simulink model "DahldissertacaoJoao"  (R2017a)
settings: Solver=ode3  StartTime=0.0  StopTime=max(Time)  FixedStep=dt  RelTol=1e-3  EnableMultiTasking=on
values from neighbouring files (symbols this model uses):
  Kw = 57.42    [maincode.m]
  Kx = 0.7682    [maincode.m]
  n = 1    [maincode.m]
  rho = 27.45    [maincode.m]
settings Model: Creator=Administrador  LastModifiedBy=vargas
settings DataIOCC: LimitDataPoints=on  SaveFormat=Array  SignalLoggingSaveFormat=ModelDataLogs
settings OptimizationCC: ExpressionDepthLimit=2147483647  LifeSpan=inf
settings DebuggingCC: UnderspecifiedInitializationDetection=Classic  MergeDetectMultiDrivingBlocksExec=none  SolverPrmCheckMsg=warning  FcnCallInpInsideContextMsg=warning  StateNameClashWarn=warning  SFUnexpectedBacktrackingDiag=warning  SFNoUnconditionalDefaultTransitionDiag=warning  SFExecutionAtInitializationDiag=none
settings HardwareCC: ProdBitPerPointer=32  ProdBitPerSizeT=32  ProdBitPerPtrDiffT=32  ProdLargestAtomicFloat=None  ProdIntDivRoundTo=Undefined  ProdEndianess=Unspecified  ProdWordSize=32  ProdHWDeviceType=32-bit Generic
settings ModelReferenceCC: PropagateSignalLabelsOutOfModel=off
settings GRTTargetCC: TargetLangStandard=C89/C90 (ANSI)  GeneratePreprocessorConditionals=Disable all  CombineOutputUpdateFcns=off  GRTInterface=on
settings ConfigComp: CovMetricSettings=dw  CovHtmlReporting=on  CovSaveCumulativeToWorkspaceVar=on  CovSaveSingleToWorkspaceVar=on  CovExternalEMLEnable=off

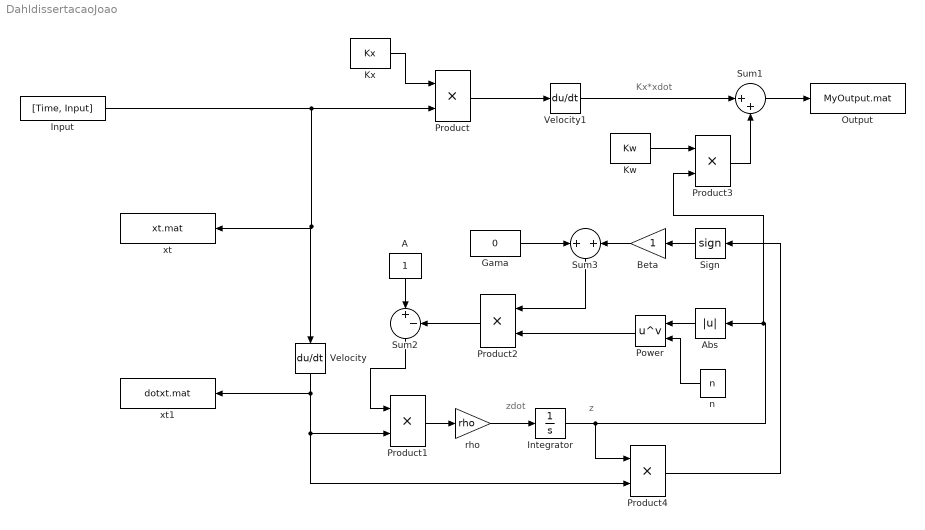
== system DahldissertacaoJoao ==
  note: Kx*xdot
  note: zdot
  note: z
  A : Constant
  Abs : Abs  SaturateOnIntegerOverflow=on
  Beta : Gain
  Gama : Constant  Value=0
  Input : FromWorkspace  VariableName=[Time, Input]  SampleTime=0
  Integrator : Integrator
  Kw : Constant  Value=Kw
  Kx : Constant  Value=Kx
  Output : ToFile  Filename=MyOutput.mat  MatrixName=MyOutput
  Power : Math  Operator=pow  SaturateOnIntegerOverflow=on
  Product{,1..4} (5 alike) : Product  RndMeth=Zero
  Sign : Signum
  Sum1 : Sum  Inputs=|++
  Sum2 : Sum  Inputs=|+-
  Sum3 : Sum  Inputs=+|+
  Velocity : Derivative
  Velocity1 : Derivative
  n : Constant  Value=n
  rho : Gain  Gain=rho
  xt : ToFile  Filename=xt.mat  MatrixName=xt
  xt1 : ToFile  Filename=dotxt.mat  MatrixName=dotxt
  wires:
  Kx/1 -> Product/1
  Abs/1 -> Power/1
  n/1 -> Power/2
  Sum1/1 -> Output/1
  Product3/1 -> Sum1/2
  Power/1 -> Product2/2
  Velocity/1 -> Product4/2, Product1/2, xt1/1
  Sum2/1 -> Product1/1
  Product4/1 -> Sign/1
  Sign/1 -> Beta/1
  Beta/1 -> Sum3/2
  Gama/1 -> Sum3/1
  Sum3/1 -> Product2/1
  A/1 -> Sum2/1
  Product2/1 -> Sum2/2
  Product1/1 -> rho/1
  rho/1 -> Integrator/1
  Product/1 -> Velocity1/1
  Velocity1/1 -> Sum1/1
  Kw/1 -> Product3/1
  Input/1 -> Velocity/1, xt/1, Product/2
  Integrator/1 -> Product4/1, Product3/2, Abs/1
